simulink model "power_quality_test"  (R2013a)
settings: Solver=ode3  StartTime=0.0  StopTime=20  FixedStep=Ts  RelTol=1e-3
values from neighbouring files (symbols this model uses):
  F4 = xlsread('F4_relay_nrel.xlsx')    [relay_settings_init.m]
  Ts = 100E-6    (= 0.0001)    [BANSHEE_init.m]    (also in Ghost_init.m)
undefined symbols (not defined in the file or in its folder): DiscIntNeverNeededParam
libraries: simulink x4, cables_lib x2, breaker_lib x2, relay_modbus_lib x2, rtio_generic_modbus x2, controllable_grid_lib x2, power_quality_lib x1, powerlib x1
settings Model: Creator=pkoralew  LastModifiedBy=pkoralew

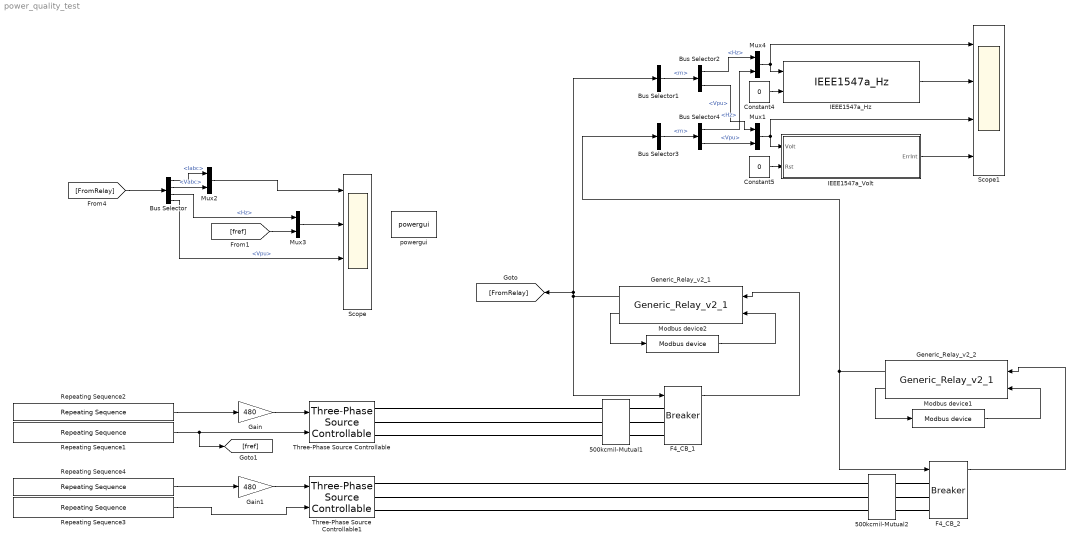
== system power_quality_test ==
  500kcmil-Mutual1 : cables_lib/500kcmil-Mutual  length=50  par_sets=1  ratio=3
  500kcmil-Mutual2 : cables_lib/500kcmil-Mutual  length=50  par_sets=1  ratio=3
  Bus Selector : BusSelector  OutputSignals=m.Iabc,m.Vabc,m.Hz,m.Vpu
  Bus Selector1 : BusSelector  OutputSignals=m
  Bus Selector2 : BusSelector  OutputSignals=Hz,Vpu
  Bus Selector3 : BusSelector  OutputSignals=m
  Bus Selector4 : BusSelector  OutputSignals=Hz,Vpu
  Constant4 : Constant  Value=0
  Constant5 : Constant  Value=0
  F4_CB_1 : breaker_lib/Breaker  Ts=Ts  mech_delay=cb_mech_delay
  F4_CB_2 : breaker_lib/Breaker  Ts=Ts  mech_delay=cb_mech_delay
  Gain : Gain  Gain=480
  Gain1 : Gain  Gain=480
  Generic_Relay_v2_1 : relay_modbus_lib/Generic_Relay_v2_1  Ts=Ts  relay_settings=[F4(2,:)]
  Generic_Relay_v2_2 : relay_modbus_lib/Generic_Relay_v2_1  Ts=Ts  relay_settings=[F4(2,:)]
  IEEE1547a_Hz : power_quality_lib/IEEE1547a_Hz
  IEEE1547a_Volt : Subsystem  AncestorBlock=power_quality_lib/IEEE1547a_Volt
  Modbus device1 : rtio_generic_modbus/Modbus device  conf_name=F4_relay_cfg1.opal  conf_name_mask=F4_relay_cfg1.xls  sample_time=Ts
  Modbus device2 : rtio_generic_modbus/Modbus device  conf_name=F4_relay_cfg1.opal  conf_name_mask=F4_relay_cfg1.xls  sample_time=Ts
  Mux{1..4} (4 alike) : Mux  Inputs=2
  Repeating Sequence1 : simulink/Sources/Repeating Sequence  rep_seq_t=[0 3 4 5 6 10 11 11.5 13 17]  rep_seq_y=[60 60 63 63 60 60 57 57 60 60]
  Repeating Sequence2 : simulink/Sources/Repeating Sequence  rep_seq_t=[0 7 7.1 7.5 8 9 9.2 10 20]  rep_seq_y=[1 1 0.1 0.1 1 1.3 1.3 1 1]
  Repeating Sequence3 : simulink/Sources/Repeating Sequence  rep_seq_t=[0 3 3.1 3.25 4 12 12.4 12.6 15 20]  rep_seq_y=[60 60 56 56 60 60 62.5 62.5 60 60]
  Repeating Sequence4 : simulink/Sources/Repeating Sequence  rep_seq_t=[0 6 6.1 6.5 8 10 10.2 11 20]  rep_seq_y=[1 1 0.6 0.6 1 1.2 1.2 1 1]
  Scope : Scope  NumInputPorts=4
      settings: YMin=-400~55.9~0.965~-1  YMax=400~57.8~1.035~1
  Scope1 : Scope  NumInputPorts=4
      settings: YMin=56~0~5.55112e-17~0  YMax=63.5~2.25~1.4~0.2  SaveName=ScopeData2  Decimation=10
  Three-Phase Source Controllable : controllable_grid_lib/Three-Phase Source Controllable
  Three-Phase Source Controllable1 : controllable_grid_lib/Three-Phase Source Controllable
  powergui : powerlib/powergui  Priority=1  SimulationMode=Discrete  SolverType=Tustin  SampleTime=100e-6  frequency=60  SPID=off  DisableSnubberDevices=off  DisableRonSwitches=off  DisableVfSwitches=off  SwTol=0  Interpol=off  DisplayEquations=off  frequencyindice=0  Pbase=100e6  ErrMax=1e-4  Iterations=50  UnitsV=kV  UnitsW=MW  FunctionMessages=off  echomessages=off  HookPort=off  EnableUseOfTLC=off  x0status=blocks  RestoreLinks=warning  ResistiveCurrentMeasurement=off  Frange=[0:2:500]  Ylog=off  Xlog=on  ShowGrid=off  save=off  variable=ZData  ZoomFFT=off  StartTime=0.0  cycles=1  DisplayStyle=1  fundamental=60  FreqAxis=off  MaxFrequency=1000  frequencyindicesteady=1  RmsSteady=1  display=off  Ts=0  methode=off
  wires:
  Repeating Sequence1/1 -> [fref], Three-Phase Source Controllable/2
  Gain/1 -> Three-Phase Source Controllable/1
  Generic_Relay_v2_1/1 -> Bus Selector1/1, [FromRelay], F4_CB_1/1
  F4_CB_1/1 -> Generic_Relay_v2_1/1
  Generic_Relay_v2_1/2 -> Modbus device2/1
  Modbus device2/1 -> Generic_Relay_v2_1/2
  [FromRelay] -> Bus Selector/1
  Bus Selector/4 -> Scope/3  "<Vpu>"
  Bus Selector/2 -> Mux2/2  "<Vabc>"
  Bus Selector/1 -> Mux2/1  "<Iabc>"
  Mux2/1 -> Scope/1
  Bus Selector/3 -> Mux3/1  "<Hz>"
  [fref] -> Mux3/2
  Mux3/1 -> Scope/2
  Bus Selector1/1 -> Bus Selector2/1  "<m>"
  Constant4/1 -> IEEE1547a_Hz/2
  Bus Selector2/2 -> Mux1/1  "<Vpu>"
  Constant5/1 -> IEEE1547a_Volt/2(Rst)
  IEEE1547a_Hz/1 -> Scope1/2
  IEEE1547a_Volt/1(ErrInt) -> Scope1/4
  Bus Selector2/1 -> Mux4/1  "<Hz>"
  Mux4/1 -> Scope1/1, IEEE1547a_Hz/1
  Repeating Sequence2/1 -> Gain/1
  Repeating Sequence3/1 -> Three-Phase Source Controllable1/2
  Gain1/1 -> Three-Phase Source Controllable1/1
  Generic_Relay_v2_2/1 -> F4_CB_2/1, Bus Selector3/1
  F4_CB_2/1 -> Generic_Relay_v2_2/1
  Generic_Relay_v2_2/2 -> Modbus device1/1
  Modbus device1/1 -> Generic_Relay_v2_2/2
  Repeating Sequence4/1 -> Gain1/1
  Bus Selector3/1 -> Bus Selector4/1  "<m>"
  Bus Selector4/1 -> Mux4/2  "<Hz>"
  Bus Selector4/2 -> Mux1/2  "<Vpu>"
  Mux1/1 -> IEEE1547a_Volt/1(Volt), Scope1/3
  connections:
  F4_CB_1/LConn2 -- 500kcmil-Mutual1/RConn2
  F4_CB_1/LConn1 -- 500kcmil-Mutual1/RConn1
  F4_CB_1/LConn3 -- 500kcmil-Mutual1/RConn3
  Three-Phase Source Controllable/RConn1 -- 500kcmil-Mutual1/LConn1
  Three-Phase Source Controllable/RConn2 -- 500kcmil-Mutual1/LConn2
  Three-Phase Source Controllable/RConn3 -- 500kcmil-Mutual1/LConn3
  F4_CB_2/LConn1 -- 500kcmil-Mutual2/RConn1
  F4_CB_2/LConn3 -- 500kcmil-Mutual2/RConn3
  F4_CB_2/LConn2 -- 500kcmil-Mutual2/RConn2
  Three-Phase Source Controllable1/RConn3 -- 500kcmil-Mutual2/LConn3
  Three-Phase Source Controllable1/RConn2 -- 500kcmil-Mutual2/LConn2
  Three-Phase Source Controllable1/RConn1 -- 500kcmil-Mutual2/LConn1

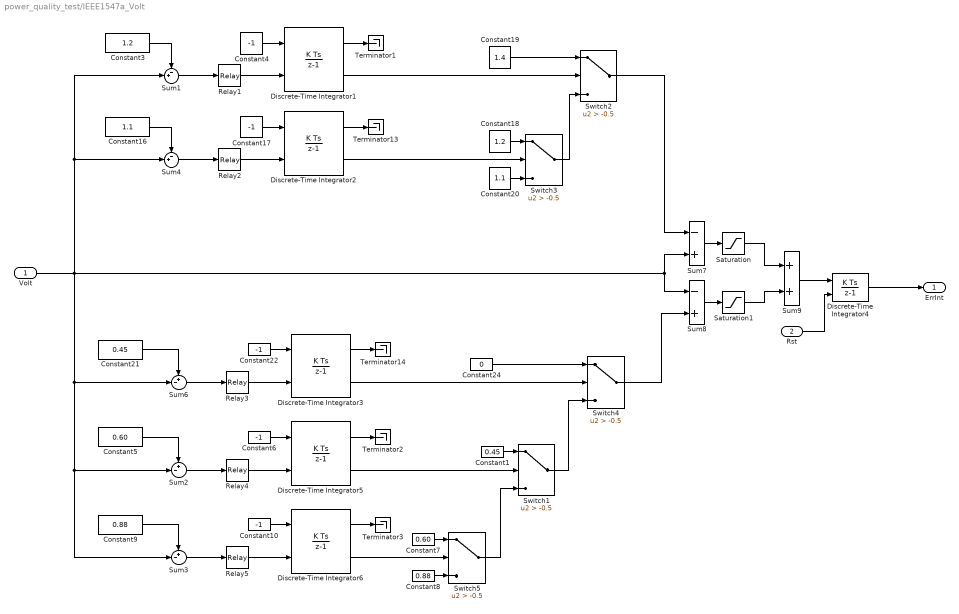
== system power_quality_test/IEEE1547a_Volt ==
  Volt : Inport
  Rst : Inport  Port=2
  Constant1 : Constant  Value=0.45
  Constant{4,6,10,17,22} (5 alike) : Constant  Value=-1
  Constant16 : Constant  Value=1.1
  Constant18 : Constant  Value=1.2
  Constant19 : Constant  Value=1.4
  Constant20 : Constant  Value=1.1
  Constant21 : Constant  Value=0.45
  Constant24 : Constant  Value=0
  Constant3 : Constant  Value=1.2
  Constant5 : Constant  Value=0.60
  Constant7 : Constant  Value=0.60
  Constant8 : Constant  Value=0.88
  Constant9 : Constant  Value=0.88
  Discrete-Time Integrator1 : DiscreteIntegrator  gainval=1  ExternalReset=rising  InitialCondition=0.16  SampleTime=Ts  LimitOutput=on  LowerSaturationLimit=0  ShowSaturationPort=on  ICPrevOutput=DiscIntNeverNeededParam  ICPrevScaledInput=DiscIntNeverNeededParam
  Discrete-Time Integrator2 : DiscreteIntegrator  gainval=1  ExternalReset=rising  InitialCondition=1  SampleTime=Ts  LimitOutput=on  LowerSaturationLimit=0  ShowSaturationPort=on  ICPrevOutput=DiscIntNeverNeededParam  ICPrevScaledInput=DiscIntNeverNeededParam
  Discrete-Time Integrator3 : DiscreteIntegrator  gainval=1  ExternalReset=rising  InitialCondition=0.16  SampleTime=Ts  LimitOutput=on  LowerSaturationLimit=0  ShowSaturationPort=on  ICPrevOutput=DiscIntNeverNeededParam  ICPrevScaledInput=DiscIntNeverNeededParam
  Discrete-Time Integrator4 : DiscreteIntegrator  gainval=1  ExternalReset=level  SampleTime=Ts  LowerSaturationLimit=0  ICPrevOutput=DiscIntNeverNeededParam  ICPrevScaledInput=DiscIntNeverNeededParam
  Discrete-Time Integrator5 : DiscreteIntegrator  gainval=1  ExternalReset=rising  InitialCondition=1  SampleTime=Ts  LimitOutput=on  LowerSaturationLimit=0  ShowSaturationPort=on  ICPrevOutput=DiscIntNeverNeededParam  ICPrevScaledInput=DiscIntNeverNeededParam
  Discrete-Time Integrator6 : DiscreteIntegrator  gainval=1  ExternalReset=rising  InitialCondition=2  SampleTime=Ts  LimitOutput=on  LowerSaturationLimit=0  ShowSaturationPort=on  ICPrevOutput=DiscIntNeverNeededParam  ICPrevScaledInput=DiscIntNeverNeededParam
  Relay{1..5} (5 alike) : Relay  OnSwitchValue=0.02  OffSwitchValue=-0.02
  Saturation : Saturate  UpperLimit=6  LowerLimit=0
  Saturation1 : Saturate  UpperLimit=6  LowerLimit=0
  Sum1 : Sum  Inputs=-+|
  Sum2 : Sum  Inputs=+-|
  Sum3 : Sum  Inputs=+-|
  Sum4 : Sum  Inputs=-+|
  Sum6 : Sum  Inputs=+-|
  Sum7 : Sum  Inputs=-+
  Sum8 : Sum  Inputs=-+
  Sum9 : Sum
  Switch{1..5} (5 alike) : Switch  Criteria=u2 > Threshold  Threshold=-0.5
  Terminator{1..3,13..14} (5 alike) : Terminator
  ErrInt : Outport
  wires:
  Volt/1 -> Sum6/2, Sum2/2, Sum3/2, Sum4/2, Sum1/2, Sum8/1, Sum7/2
  Constant9/1 -> Sum3/1
  Sum3/1 -> Relay5/1
  Discrete-Time Integrator6/1 -> Terminator3/1
  Relay5/1 -> Discrete-Time Integrator6/2
  Constant10/1 -> Discrete-Time Integrator6/1
  Discrete-Time Integrator6/2 -> Switch5/2
  Constant8/1 -> Switch5/3
  Constant7/1 -> Switch5/1
  Saturation/1 -> Sum9/1
  Saturation1/1 -> Sum9/2
  Constant5/1 -> Sum2/1
  Sum2/1 -> Relay4/1
  Discrete-Time Integrator5/1 -> Terminator2/1
  Relay4/1 -> Discrete-Time Integrator5/2
  Constant6/1 -> Discrete-Time Integrator5/1
  Constant3/1 -> Sum1/1
  Sum1/1 -> Relay1/1
  Relay1/1 -> Discrete-Time Integrator1/2
  Discrete-Time Integrator1/1 -> Terminator1/1
  Constant4/1 -> Discrete-Time Integrator1/1
  Discrete-Time Integrator5/2 -> Switch1/2
  Switch5/1 -> Switch1/3
  Constant1/1 -> Switch1/1
  Constant21/1 -> Sum6/1
  Sum6/1 -> Relay3/1
  Discrete-Time Integrator3/2 -> Switch4/2
  Discrete-Time Integrator3/1 -> Terminator14/1
  Relay3/1 -> Discrete-Time Integrator3/2
  Constant24/1 -> Switch4/1
  Constant22/1 -> Discrete-Time Integrator3/1
  Switch1/1 -> Switch4/3
  Constant19/1 -> Switch2/1
  Constant18/1 -> Switch3/1
  Switch3/1 -> Switch2/3
  Discrete-Time Integrator1/2 -> Switch2/2
  Discrete-Time Integrator2/2 -> Switch3/2
  Constant20/1 -> Switch3/3
  Discrete-Time Integrator4/1 -> ErrInt/1
  Sum8/1 -> Saturation1/1
  Rst/1 -> Discrete-Time Integrator4/2
  Sum7/1 -> Saturation/1
  Switch4/1 -> Sum8/2
  Switch2/1 -> Sum7/1
  Sum9/1 -> Discrete-Time Integrator4/1
  Constant16/1 -> Sum4/1
  Sum4/1 -> Relay2/1
  Relay2/1 -> Discrete-Time Integrator2/2
  Discrete-Time Integrator2/1 -> Terminator13/1
  Constant17/1 -> Discrete-Time Integrator2/1
